simulink model "prelab3_part7"  (R2021b)
settings: Solver=VariableStepAuto  StartTime=0.0  StopTime=10.0  RelTol=1e-3
settings Model: Creator=golmehr  LastModifiedBy=mahya
settings SolverCC: AlgebraicLoopSolver=TrustRegion
settings DataIOCC: ReturnWorkspaceOutputs=off
settings DebuggingCC: SFMachineParentedDataDiag=warning  ArithmeticOperatorsInVariantConditions=warning
settings SFSimCC: CustomCodeUndefinedFunction=UseInterfaceOnly

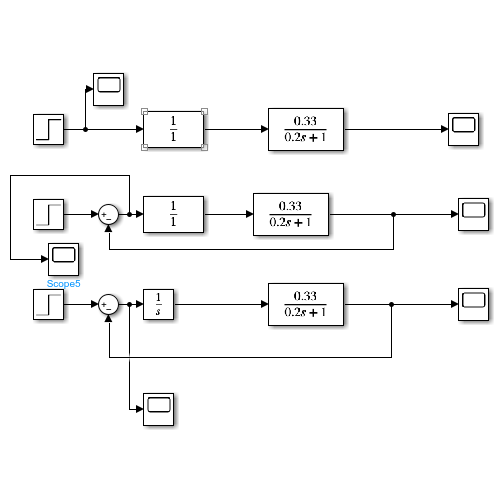
[thumbnail: Simulink's stored preview of the top-level diagram]
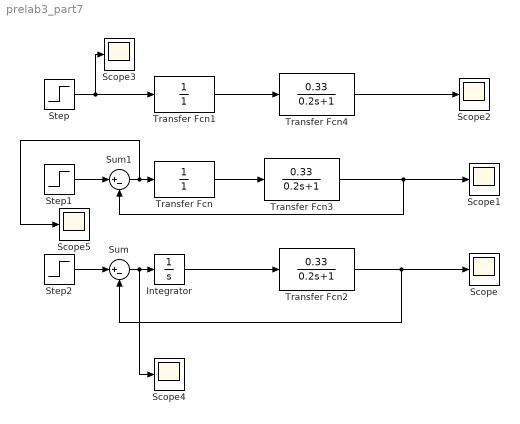
== system prelab3_part7 ==
  Integrator : Integrator
  Scope{,1..5} (6 alike) : Scope
  Step : Step  Time=0  SampleTime=0
  Step1 : Step  Time=0  SampleTime=0
  Step2 : Step  Time=0  SampleTime=0
  Sum : Sum  Inputs=|+-
  Sum1 : Sum  Inputs=|+-
  Transfer Fcn : TransferFcn  Denominator=[1]
  Transfer Fcn1 : TransferFcn  Denominator=[1]
  Transfer Fcn2 : TransferFcn  Numerator=[0.33]  Denominator=[0.2 1]
  Transfer Fcn3 : TransferFcn  Numerator=[0.33]  Denominator=[0.2 1]
  Transfer Fcn4 : TransferFcn  Numerator=[0.33]  Denominator=[0.2 1]
  wires:
  Step/1 -> Scope3/1, Transfer Fcn1/1
  Integrator/1 -> Transfer Fcn2/1
  Transfer Fcn2/1 -> Sum/2, Scope/1
  Sum/1 -> Scope4/1, Integrator/1
  Step2/1 -> Sum/1
  Transfer Fcn/1 -> Transfer Fcn3/1
  Transfer Fcn3/1 -> Sum1/2, Scope1/1
  Sum1/1 -> Scope5/1, Transfer Fcn/1
  Step1/1 -> Sum1/1
  Transfer Fcn1/1 -> Transfer Fcn4/1
  Transfer Fcn4/1 -> Scope2/1
